simulink model "nonlinear_mpc_controller"  (R2025a)
settings: Solver=FixedStepAuto  StartTime=0.0  StopTime=10.0  RelTol=1e-3
undefined symbols (not defined in the file): A, B, p_btheta, p_bx, p_g, p_G, p_Iw, p_Jp, p_Ke, p_Kt, p_l, p_La, p_M, p_m, p_r, p_Ra
libraries: eeLuenbergerObserver x1, mpclib x1
settings Model: Creator=nopla  LastModifiedBy=nopla
settings OptimizationCC: UseDivisionForNetSlopeComputation=on

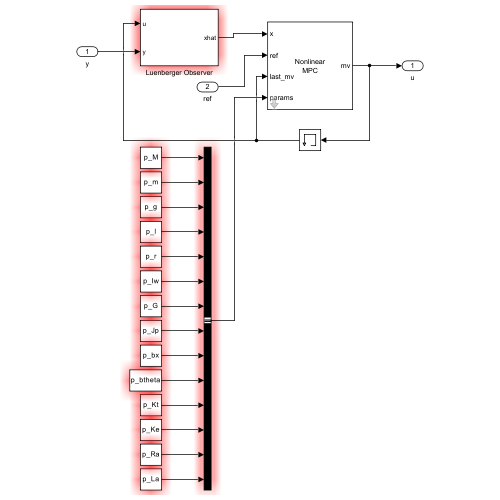
[thumbnail: Simulink's stored preview of the top-level diagram]
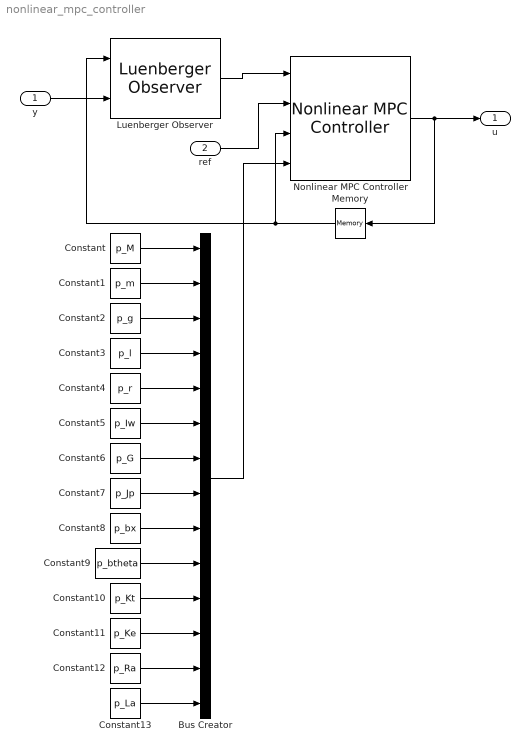
== system nonlinear_mpc_controller ==
  y : Inport  PortDimensions=[2; 1]
  ref : Inport  Port=2  PortDimensions=[1; 2]
  Bus Creator : BusCreator  Inputs=14  OutDataTypeStr=Bus: ParamsBus
      settings: InheritFromInputs=off
  Constant : Constant  Value=p_M
  Constant1 : Constant  Value=p_m
  Constant10 : Constant  Value=p_Kt
  Constant11 : Constant  Value=p_Ke
  Constant12 : Constant  Value=p_Ra
  Constant13 : Constant  Value=p_La
  Constant2 : Constant  Value=p_g
  Constant3 : Constant  Value=p_l
  Constant4 : Constant  Value=p_r
  Constant5 : Constant  Value=p_Iw
  Constant6 : Constant  Value=p_G
  Constant7 : Constant  Value=p_Jp
  Constant8 : Constant  Value=p_bx
  Constant9 : Constant  Value=p_btheta
  Luenberger Observer : eeLuenbergerObserver/Luenberger Observer  StateSpaceType=Continuous-time  Ad=1  Bd=1  Cd=1  Dd=1  A=A  B=B  C=[1 0 0 0 0; 0 0 1 0 0]  D=[0; 0]  ObserverDesign=Desired eigenvalues  Ld=1  DesiredEigenvalues=observer_target_eigenvalues  x0=[0; 0; 0; 0; 0]  Tsd=0.1  Ts=0.001
      settings: LibrarySourceBlock=ee_sl_lib/Observers/Luenberger Observer
  Memory : Memory
  Nonlinear MPC Controller : mpclib/Nonlinear MPC Controller  nlmpcobj=nlmpcobj  UseObjectTs=on  UseMEX=off  md_enabled=off  mvtarget_enabled=off  param_enabled=on  cost_enabled=off  mvseq_enabled=off  stateseq_enabled=off  ovseq_enabled=off  slack_enabled=off  status_enabled=off  ov_min=off  ov_max=off  mv_min=off  mv_max=off  mvrate_min=off  mvrate_max=off  state_min=off  state_max=off  ov_weight=off  mv_weight=off  mvrate_weight=off  ecr_weight=off  nlp_initialize=off
  u : Outport
  wires:
  Nonlinear MPC Controller/1 -> Memory/1, u/1
  y/1 -> Luenberger Observer/2
  Memory/1 -> Luenberger Observer/1, Nonlinear MPC Controller/3
  Luenberger Observer/1 -> Nonlinear MPC Controller/1
  ref/1 -> Nonlinear MPC Controller/2
  Bus Creator/1 -> Nonlinear MPC Controller/4
  Constant/1 -> Bus Creator/1
  Constant1/1 -> Bus Creator/2
  Constant2/1 -> Bus Creator/3
  Constant3/1 -> Bus Creator/4
  Constant6/1 -> Bus Creator/7
  Constant7/1 -> Bus Creator/8
  Constant4/1 -> Bus Creator/5
  Constant5/1 -> Bus Creator/6
  Constant10/1 -> Bus Creator/11
  Constant11/1 -> Bus Creator/12
  Constant8/1 -> Bus Creator/9
  Constant9/1 -> Bus Creator/10
  Constant12/1 -> Bus Creator/13
  Constant13/1 -> Bus Creator/14
